simulink model "Task3_Numerical_Stability"  (R2019b)
settings: Solver=FixedStepAuto  StartTime=0.0  StopTime=100  FixedStep=0.01  RelTol=1e-3
settings Model: Creator=Marco Nugnes  LastModifiedBy=Davide

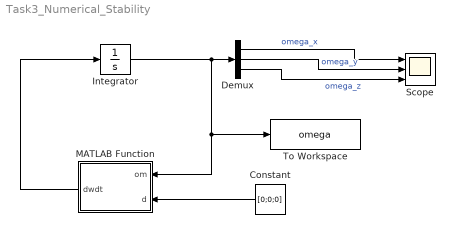
== system Task3_Numerical_Stability ==
  Constant : Constant  Value=[0;0;0]
  Demux : Demux  Outputs=3
  Integrator : Integrator  InitialCondition=[0; 0; 2*pi]
  MATLAB Function : MATLAB Function  TreatAsAtomicUnit=on
  Scope : Scope  NumInputPorts=3
  To Workspace : ToWorkspace  VariableName=omega  SampleTime=-1
  wires:
  Integrator/1 -> To Workspace/1, MATLAB Function/1(om), Demux/1
  Demux/1 -> Scope/1  "omega_x"
  Demux/2 -> Scope/2  "omega_y"
  Demux/3 -> Scope/3  "omega_z"
  MATLAB Function/1(dwdt) -> Integrator/1
  Constant/1 -> MATLAB Function/2(d)

== matlab function Task3_Numerical_Stability/MATLAB Function ==
  data: om input; dwdt output; d input
function dwdt = euler_eq(om,d)

% Angular velocities
wx = om(1);
wy = om(2);
wz = om(3);

% Definition of the inertia moments
Ix = 0.01;                    
Iy = 0.05;
%Iy = 0.08; % to be used with 0 disturbances and perturbed initial condition
Iz = 0.07;

% Perturbed initial condition
%[0+0.001; 0+0.001; 2*pi+0.001] 

% Inertia Ratio
kx = (Iy-Iz)/Ix;
ky = (Iz-Ix)/Iy;
kz = (Ix-Iy)/Iz;

% Euler equations
dwxdt = kx*wy*wz + d(1)/Ix;
dwydt = ky*wx*wz + d(2)/Iy;
dwzdt = kz*wx*wy + d(3)/Iz;

dwdt = [dwxdt;dwydt;dwzdt];
